simulink model "model"  (R2023a)
settings: Solver=VariableStepAuto  StartTime=0.0  StopTime=10.0  RelTol=1e-3
settings Model: Creator=Theomur  LastModifiedBy=пользователь

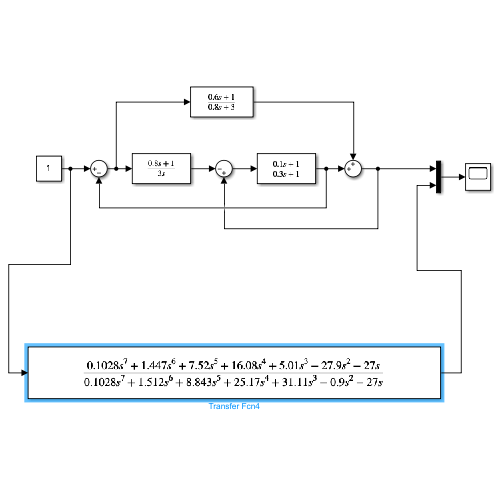
[thumbnail: Simulink's stored preview of the top-level diagram]
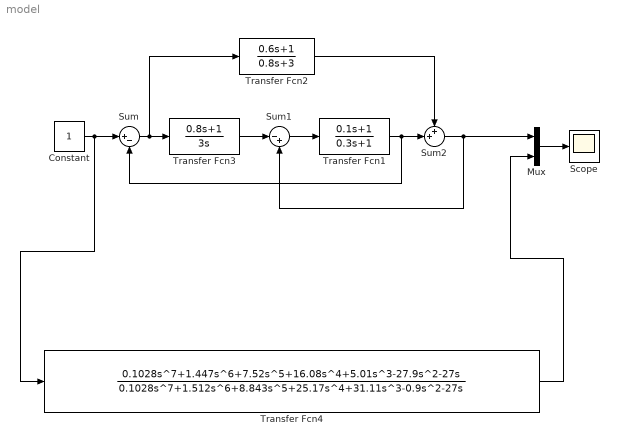
== system model ==
  Constant : Constant
  Mux : Mux  Inputs=2
  Scope : Scope
  Sum : Sum  Inputs=|+-
  Sum1 : Sum  Inputs=|-+
  Sum2 : Sum  Inputs=++|
  Transfer Fcn1 : TransferFcn  Numerator=[0.1 1]  Denominator=[0.3 1]
  Transfer Fcn2 : TransferFcn  Numerator=[0.6 1]  Denominator=[0.8 3]
  Transfer Fcn3 : TransferFcn  Numerator=[0.8 1]  Denominator=[3 0]
  Transfer Fcn4 : TransferFcn  Numerator="[  0.1028 1.447 7.52 16.08 5.01 -27.9 -27 0]"  Denominator="[  0.1028 1.512 8.843 25.17 31.11 -0.9 -27 0]"
  wires:
  Constant/1 -> Transfer Fcn4/1, Sum/1
  Sum/1 -> Transfer Fcn3/1, Transfer Fcn2/1
  Transfer Fcn3/1 -> Sum1/1
  Sum1/1 -> Transfer Fcn1/1
  Transfer Fcn1/1 -> Sum/2, Sum2/2
  Sum2/1 -> Mux/1, Sum1/2
  Transfer Fcn2/1 -> Sum2/1
  Mux/1 -> Scope/1
  Transfer Fcn4/1 -> Mux/2
